simulink library "MultiModelToolbox"  (R2024b)
settings: Solver=VariableStepAuto  StartTime=0.0  StopTime=10.0  RelTol=1e-3
undefined symbols (not defined in the file): A, B, C, D, gravitationalAcceleration, MotorTorqueMax, roadB, roadC, roadD, roadE, roadSlope, stateSpace, Ts
libraries: $bdroot x5, autolibshared x1
settings Model: Creator=jdazo054  LastModifiedBy=jdazo054

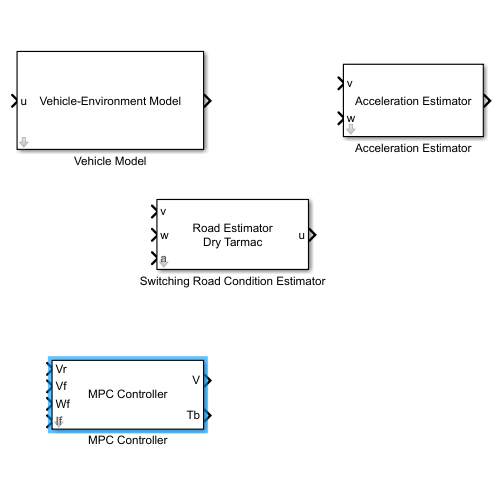
[thumbnail: Simulink's stored preview of the top-level diagram]
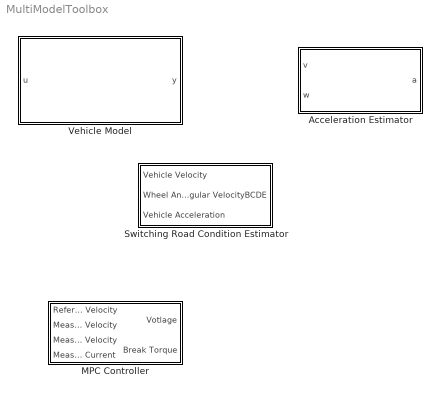
== system MultiModelToolbox ==
  Acceleration Estimator : Subsystem  mask{RoadCondition=Dry Tarmac, vehicleMass=1500, wheelInertia=0.8, wheelRadius=0.3, motorInertia=1, motorTorqueConstant=5, Clambda=0}
      mask prompts: RoadCondition "Road Condition"; vehicleMass "Vehicle Mass"; wheelInertia "Wheel Inertia"; wheelRadius "Wheel Radius"; motorInertia "Axle Inertia"; motorTorqueConstant "Torque Constant"
      mask TypeOptions RoadCondition: Dry Tarmac | Wet Tarmac | Snow | Ice
      mask DialogControl DescGroupVar Prompt: Acceleration Estimator
      mask DialogControl DescTextVar Prompt: This subsystem estimates vehicle acceleration using a linearized Pacejka tire model and Newton’s second law. Tire force is computed based on the selected road condition, which determines the Pacejka coefficients. The estimated force is divided by the user-defined vehicle mass to calculate acceleration. Road friction effects are implicitly modeled through the road type parameter.
      mask DialogControl RoadCondition Tooltip: Road surface type (affects traction and friction). Selects the corresponding coefficients (B, C, D, E) for the Pacejka Magic Formula used to compute linearized tire stiffness (Clambda). Options: Dry Tarmac, Wet Tarmac, Snow, Ice.
      mask DialogControl Container3 Prompt: Vehicle Parameters
      mask DialogControl vehicleMass Tooltip: Mass of the vehicle in kilograms (kg).
      mask DialogControl wheelInertia Tooltip: Moment of inertia of the wheel in kg·m².
      mask DialogControl wheelRadius Tooltip: Radius of the wheel in meters (m).
      mask DialogControl Container4 Prompt: Motor Parameters
      mask DialogControl motorInertia Tooltip: Moment of inertia of the motor rotor in kg·m².
      mask DialogControl motorTorqueConstant Tooltip: Motor torque constant in newton-meters per ampere (Nm/A).
      mask DialogControl Container5 Prompt: Invisible Parameters
      mask Display:
      | disp('Acceleration Estimator');
      | port_label('input', 1, 'v');
      | port_label('input', 2, 'w');
  MPC Controller : Subsystem  mask{Parameter1=0, stateSpace=stateSpace}
      mask prompts: Parameter1 "Prediction Horizon"
      mask DialogControl DescGroupVar Prompt: EV Model Predictive Controller
      mask DialogControl DescTextVar Prompt: This block implements a discrete-time linear Model Predictive Control (MPC) for set-point tracking of a 3-state, 1-input system.
      mask Display:
      | disp('MPC Controller');
      | port_label('input', 1, 'Vr');
      | port_label('input', 2, 'Vf');
      | port_label('input', 3, 'Wf');
      | port_label('input', 4, 'If');
      | port_label('output', 1, 'V');
      | port_label('output', 2, 'Tb');
  Switching Road Condition Estimator : Subsystem  mask{currentRoadIdx=1}
      mask Display:
      | % Display title
      | disp('Road Estimator\n');
      | 
      | currentRoadIdx = get_param(gcb, "currentRoadIdx");
      | 
      | % Display road label (use variable stored in mask or workspace)
      | switch currentRoadIdx
      |     case '1'
      |         disp('\nDry Tarmac');
      |     case '2'
      |         disp('\nWet Tarmac');
      |     case '3'
      |         disp('\nSnow');
      |     case '4'
      |         disp('\nIce');
      |     otherwise
      |         disp("\nUnknown");
      | end
      | port_label('input', 1, 'v');
      | port_label('input', 2, 'w');
      | port_label('input', 3, 'a');
      | port_label('output', 1, 'u');
  Vehicle Model : Subsystem  mask{RoadCondition=Dry Tarmac, vehicleMass=1500, wheelInertia=0.8, wheelRadius=0.3, motorInertia=1, motorResistance=0.1, motorTorqueConstant=5, motorInductance=0.005, motorBackEMFConstant=0.004, A_matrix=0, B_matrix=0, C_matrix=0, D_matrix=0}
      mask prompts: RoadCondition "Road Condition"; vehicleMass "Vehicle Mass"; wheelInertia "Wheel Inertia"; wheelRadius "Wheel Radius"; motorInertia "Axle Inertia"; motorResistance "Armature Resistance"; motorTorqueConstant "Torque Constant"; motorInductance "Armature Inductance"; motorBackEMFConstant "Armature EMF Constant"
      mask TypeOptions RoadCondition: Dry Tarmac | Wet Tarmac | Snow | Ice
      mask DialogControl DescGroupVar Prompt: Vehicle-Environment Model
      mask DialogControl DescTextVar Prompt: MATLAB/SIMULINK Model of a Vehicle. Designed for Longitudinal Road Friction Adaptive Control using Multi-Model Adaptive Estimators (MMAEs)
      mask DialogControl RoadCondition Tooltip: Road surface type (affects traction and friction). Selects the corresponding coefficients (B, C, D, E) for the Pacejka Magic Formula used to compute linearized tire stiffness (Clambda). Options: Dry Tarmac, Wet Tarmac, Snow, Ice.
      mask DialogControl Container3 Prompt: Vehicle Parameters
      mask DialogControl vehicleMass Tooltip: Mass of the vehicle in kilograms (kg).
      mask DialogControl wheelInertia Tooltip: Moment of inertia of the wheel in kg·m².
      mask DialogControl wheelRadius Tooltip: Radius of the wheel in meters (m).
      mask DialogControl Container4 Prompt: Motor Parameters
      mask DialogControl motorInertia Tooltip: Moment of inertia of the motor rotor in kg·m².
      mask DialogControl motorResistance Tooltip: Electrical resistance of the motor windings in ohms (Ω).
      mask DialogControl motorTorqueConstant Tooltip: Motor torque constant in newton-meters per ampere (Nm/A).
      mask DialogControl motorInductance Tooltip: Electrical inductance of the motor windings in henries (H).
      mask DialogControl motorBackEMFConstant Tooltip: Motor back EMF constant in volts per radian per second (V·s/rad).
      mask Display:
      | disp('Vehicle-Environment Model');
      | port_label('input', 1, 'u');

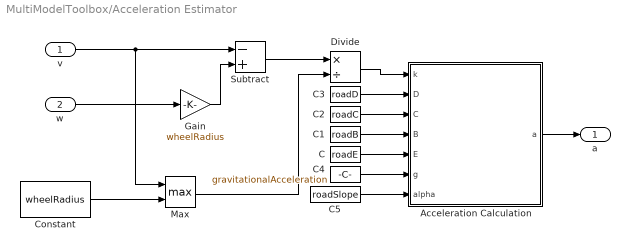
== system MultiModelToolbox/Acceleration Estimator ==
  v : Inport
  w : Inport  Port=2
  Acceleration Calculation : MATLAB Function  TreatAsAtomicUnit=on
  C : Constant  Value=roadE
  C1 : Constant  Value=roadB
  C2 : Constant  Value=roadC
  C3 : Constant  Value=roadD
  C4 : Constant  Value=gravitationalAcceleration
  C5 : Constant  Value=roadSlope
  Constant : Constant  Value=wheelRadius
  Divide : Product  Inputs=*/
  Gain : Gain  Gain=wheelRadius
  Max : MinMax  Function=max  Inputs=2
  Subtract : Sum  Inputs=-+
  a : Outport
  wires:
  Constant/1 -> Max/2
  v/1 -> Max/1, Subtract/1
  w/1 -> Gain/1
  Gain/1 -> Subtract/2
  Subtract/1 -> Divide/1
  Max/1 -> Divide/2
  Divide/1 -> Acceleration Calculation/1(k)
  C3/1 -> Acceleration Calculation/2(D)
  C2/1 -> Acceleration Calculation/3(C)
  C1/1 -> Acceleration Calculation/4(B)
  C/1 -> Acceleration Calculation/5(E)
  C4/1 -> Acceleration Calculation/6(g)
  C5/1 -> Acceleration Calculation/7(alpha)
  Acceleration Calculation/1(a) -> a/1

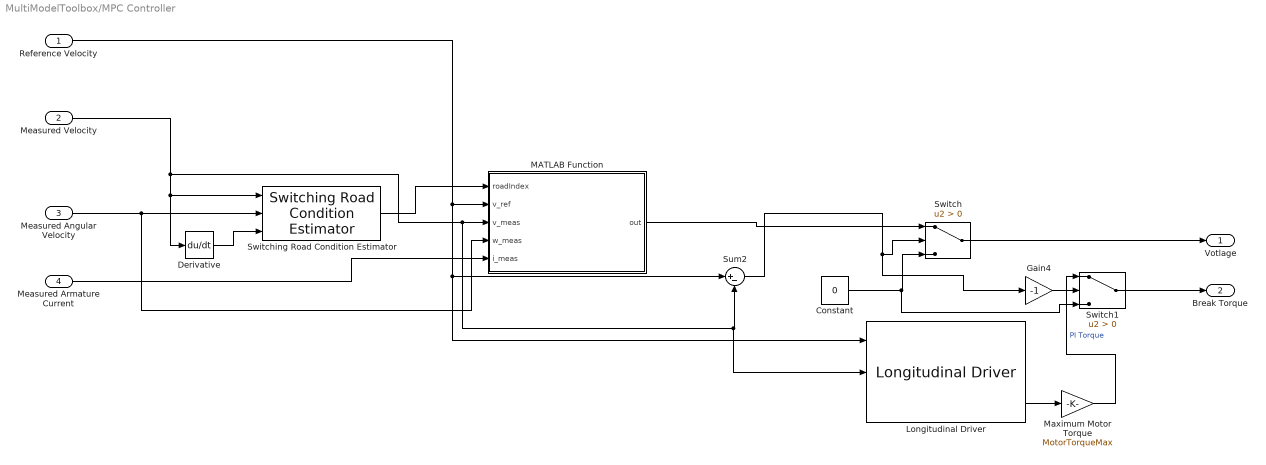
== system MultiModelToolbox/MPC Controller ==
  Reference Velocity : Inport
  Measured Velocity : Inport  Port=2
  Measured Angular Velocity : Inport  Port=3
  Measured Armature Current : Inport  Port=4
  Constant : Constant  Value=0
  Derivative : Derivative
  Gain4 : Gain  Gain=-1
  Longitudinal Driver : autolibshared/Longitudinal Driver  extAccelOvr=off  extDecelOvr=off  extAccelHld=off  extDecelHld=off  extAccelZero=off  extDecelZero=off  cntrlType=PI  shftType=None  velUnits=m/s  gearOut=off  Kp=8  Ki=2  Kff=.1  Kg=0  VehVelVec=[0 100]  KffVec=[.1 .1]  KpVec=[10 10]  KiVec=[5 5]  KgVec=[0 0]  m=1500  Kpt=3000  tau=.1  L=2  aR=200  bR=2.5  cR=.5  g=9.81  vnom=5  Kaw=1  tauerr=.01  tauPt=2  GearInit=0  tShift=.1  pdlVec=[0.1 0.4 0.5 0.9]  upShftTbl=[-1 12.9375 26.4375 39.9375 51.18749999999999 62.4375 72.84375 83.25;-1 16.3125 29.8125 43.3125 54.5624 65.8125 76.78125 87.75;-1 19.6875 33.1875 46.68749999999999 57.9375 69.1875 80.71875 92.25;-1 33 52.5 77.25 100.5 138.75 161.875 185]  dwnShftTbl=[1 9.5625 23.0625 36.5625 47.8125 59.0625 68.90625 78.75;1 12.9375 26.4375 39.9375 51.18749999999999 62.4375 72.84375 83.25;1 16.3125 29.8125 43.3125 54.562499 65.8125 76.78125 87.75;1 19.6875 33.1875 46.68749999999999 57.9375 69.1875 80.71875 92.25]  tClutch=.5  tRev=.5  tPark=120  aMode=2  UpGearVec="[0  1  2  3  4  5  6  7]"  DownGearVec="[1  2  3  4  5  6  7  8]"
      settings: LibrarySourceBlock=vehdynlibdriver/Longitudinal Driver
  MATLAB Function : MATLAB Function  TreatAsAtomicUnit=on  SystemSampleTime=Ts
  Maximum Motor Torque : Gain  Gain=MotorTorqueMax
  Sum2 : Sum  Inputs=|+-
  Switch : Switch  Criteria=u2 > Threshold  SaturateOnIntegerOverflow=off  InputSameDT=off
  Switch1 : Switch  Criteria=u2 > Threshold  SaturateOnIntegerOverflow=off  InputSameDT=off
  Switching Road Condition Estimator : $bdroot/Switching Road Condition Estimator  currentRoadIdx=1
  Votlage : Outport
  Break Torque : Outport  Port=2
  wires:
  Reference Velocity/1 -> Longitudinal Driver/1, Sum2/1, MATLAB Function/2(v_ref)
  Measured Angular Velocity/1 -> MATLAB Function/4(w_meas), Switching Road Condition Estimator/2
  Measured Velocity/1 -> Longitudinal Driver/2, Sum2/2, MATLAB Function/3(v_meas), Derivative/1, Switching Road Condition Estimator/1
  Switching Road Condition Estimator/1 -> MATLAB Function/1(roadIndex)
  Derivative/1 -> Switching Road Condition Estimator/3
  MATLAB Function/1(out) -> Switch/1
  Measured Armature Current/1 -> MATLAB Function/5(i_meas)
  Switch/1 -> Votlage/1
  Longitudinal Driver/3 -> Maximum Motor Torque/1
  Constant/1 -> Switch1/3, Switch/3
  Maximum Motor Torque/1 -> Switch1/1  "PI Torque"
  Sum2/1 -> Gain4/1, Switch/2
  Gain4/1 -> Switch1/2
  Switch1/1 -> Break Torque/1

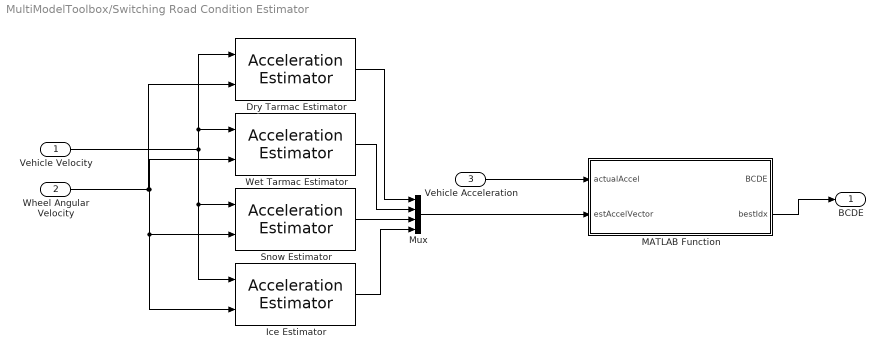
== system MultiModelToolbox/Switching Road Condition Estimator ==
  Vehicle Velocity : Inport
  Wheel Angular Velocity : Inport  Port=2
  Vehicle Acceleration : Inport  Port=3
  Dry Tarmac Estimator : $bdroot/Acceleration Estimator  RoadCondition=Dry Tarmac  vehicleMass=1500  wheelInertia=0.8  wheelRadius=0.3  motorInertia=1  motorTorqueConstant=5  Clambda=0
      link override Acceleration Calculation: SystemSampleTime=-1
  Ice Estimator : $bdroot/Acceleration Estimator  RoadCondition=Ice  vehicleMass=1500  wheelInertia=0.8  wheelRadius=0.3  motorInertia=1  motorTorqueConstant=5  Clambda=0
  MATLAB Function : MATLAB Function  TreatAsAtomicUnit=on
  Mux : Mux
  Snow Estimator : $bdroot/Acceleration Estimator  RoadCondition=Snow  vehicleMass=1500  wheelInertia=0.8  wheelRadius=0.3  motorInertia=1  motorTorqueConstant=5  Clambda=0
  Wet Tarmac Estimator : $bdroot/Acceleration Estimator  RoadCondition=Wet Tarmac  vehicleMass=1500  wheelInertia=0.8  wheelRadius=0.3  motorInertia=1  motorTorqueConstant=5  Clambda=0
  BCDE : Outport
  wires:
  Vehicle Velocity/1 -> Ice Estimator/1, Snow Estimator/1, Dry Tarmac Estimator/1, Wet Tarmac Estimator/1
  Wheel Angular Velocity/1 -> Ice Estimator/2, Snow Estimator/2, Wet Tarmac Estimator/2, Dry Tarmac Estimator/2
  Dry Tarmac Estimator/1 -> Mux/1
  Wet Tarmac Estimator/1 -> Mux/2
  Snow Estimator/1 -> Mux/3
  Ice Estimator/1 -> Mux/4
  Mux/1 -> MATLAB Function/2(estAccelVector)
  Vehicle Acceleration/1 -> MATLAB Function/1(actualAccel)
  MATLAB Function/2(bestIdx) -> BCDE/1

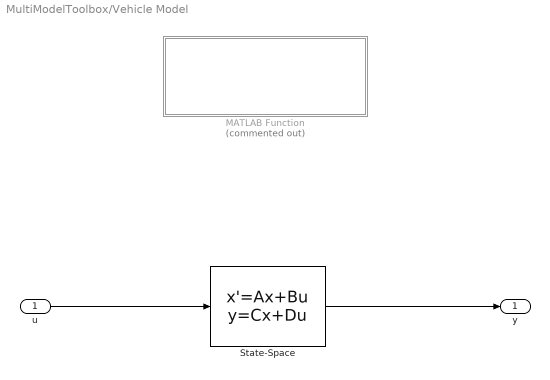
== system MultiModelToolbox/Vehicle Model ==
  u : Inport
  MATLAB Function : MATLAB Function  Commented=on  TreatAsAtomicUnit=on
  State-Space : StateSpace  A=A_matrix  B=B_matrix  C=C_matrix  D=D_matrix  InitialCondition=0
  y : Outport
  wires:
  u/1 -> State-Space/1
  State-Space/1 -> y/1

== matlab function MultiModelToolbox/Acceleration Estimator/Acceleration Calculation ==
  data: k input; a output; D input; C input; B input; E input; g input; alpha input
function a = PacejkaFormula(k, D, C, B, E, g, alpha)
    
    % Compute acceleration
    num_wheels = 2;
    ux = D * sin(C * atan(B * k - E * (B * k - atan(B * k))));
    a = num_wheels * 1 * cos(alpha) * ux;

== matlab function MultiModelToolbox/Vehicle Model/MATLAB Function ==
  data: B parameter; C parameter; D parameter; A parameter
function GenerateStateSpaceMatrices(B, C, D, A)
%#codegen

% Get parameters from the block mask
roadCondition        = get_param(gcb, 'RoadCondition'); % e.g. 'Dry Tarmac'
vehicleMass          = str2double(get_param(gcb, 'vehicleMass'));         
wheelInertia         = str2double(get_param(gcb, 'wheelInertia'));        
wheelRadius          = str2double(get_param(gcb, 'wheelRadius'));         
motorInertia         = str2double(get_param(gcb, 'motorInertia'));        
motorResistance      = str2double(get_param(gcb, 'motorResistance'));     
motorInductance      = str2double(get_param(gcb, 'motorInductance'));     
motorTorqueConstant  = str2double(get_param(gcb, 'motorTorqueConstant')); 
motorBackEMFConstant = str2double(get_param(gcb, 'motorBackEMFConstant'));

% Gravity constant
g = 9.81;

% Set Magic Formula Coefficients based on Road Condition    
switch roadCondition
    case 'Dry Tarmac'
        roadB = 10; roadC = 1.9; roadD = 1; roadE = 0.97;
    case 'Wet Tarmac'
        roadB = 12; roadC = 2.3; roadD = 0.82; roadE = 1;
    case 'Snow'
        roadB = 5;  roadC = 2;   roadD = 0.3;  roadE = 1;
    case 'Ice'
        roadB = 4;  roadC = 2;   roadD = 0.1;  roadE = 1;
    otherwise
        roadB = 10; roadC = 1.9; roadD = 1; roadE = 0.97;
end

% Compute linearized slip stiffness based of the derivative
Clambda = roadB*roadC*roadD

A = [
    (- 4* Clambda * gravitationalAcceleration * cos(roadSlope)) / wheelRadius - C1 / vehicleMass, 4*Clambda * gravitationalAcceleration * cos(roadSlope), 0;
    (4*Clambda * gravitationalAcceleration * cos(roadSlope)) / (motorInertia + wheelInertia), - (4*Clambda * wheelRadius * vehicleMass * gravitationalAcceleration * cos(roadSlope)) / (motorInertia + wheelInertia), motorTorqueConstant / (motorInertia + wheelInertia);
    0, -motorBackEMFConstant / motorInductance, -motorResistance / motorInductance
];

% Define B matrix with input voltage (Vin)
B = [
    0;
    0;
    1 / motorInductance
];

% Output matrix (only velocity is measured)
C = [1 0 0]; 
D = 0;

== matlab function MultiModelToolbox/Switching Road Condition Estimator/MATLAB Function ==
  settings: updateMethod=DISCRETE
  data: actualAccel input; BCDE output; estAccelVector input; bestIdx output
function [BCDE, bestIdx] = fcn(actualAccel, estAccelVector)
% Inputs:
%   actualAccel     - scalar (latest measured acceleration)
%   estAccelVector  - 4×1 vector (latest estimated acceleration for each road condition)
% Outputs:
%   BCDE            - 1×4 vector: [B C D E] for best-fit road
%   bestIdx         - integer: index of best-fit road condition

    % --- Parameters ---
    windowSize = 1000;  % Moving average window size (adjustable)

    % Define road surface Pacejka parameters: [B C D E]
    params = [
        10, 1.9, 1.00, 0.97;  % Dry
        12, 2.3, 0.82, 1.00;  % Wet
        5,  2.0, 0.30, 1.00;  % Snow
        4,  2.0, 0.10, 1.00   % Ice
    ];

    numConditions = size(params, 1);

    % --- Persistent Error History Buffer ---
    persistent errHist
    if isempty(errHist)
        errHist = zeros(numConditions, windowSize);
    end

    % --- Update Buffer with New Squared Errors ---
    for i = 1:numConditions
        %fprintf("Road Condition: %d", i);
        err = actualAccel - estAccelVector(i);
        %fprintf("Error: %d", err);
        errHist(i, :) = [errHist(i, 2:end), err^2];  % Shift left, append new
    end

    % --- Compute Smoothed Error (Moving Average) ---
    avgError = mean(errHist, 2);  % 4×1 vector

    % --- Find Best Matching Road Condition ---
    [~, bestIdx] = min(avgError);
    BCDE = params(bestIdx, :);
end

== matlab function MultiModelToolbox/MPC Controller/MATLAB Function ==
  data: roadIndex input; out output; v_ref input; v_meas input; w_meas input; i_meas input; stateSpace parameter
function out = lmpc_step(roadIndex, v_ref, v_meas, w_meas, i_meas, stateSpace)
% LMPC_STEP  One-step linear MPC with condensed QP formulation.
% Inputs:
%   roadIndex : integer in {1=dry, 2=wet, 3=snow, 4=ice}
%   v_ref     : current reference velocity [m/s] (assumed constant over horizon)
%   v_meas    : measured vehicle velocity [m/s]
%

    %===========================================================
    % 0) MPC Controller Parameter Definition
    %===========================================================

    switch roadIndex
        case 1
            A_matrix = stateSpace.dry_tarmac.A;
            B_matrix = stateSpace.dry_tarmac.B;
        case 2
            A_matrix = stateSpace.wet_tarmac.A;
            B_matrix = stateSpace.wet_tarmac.B;
        case 3
            A_matrix = stateSpace.snow.A;
            B_matrix = stateSpace.snow.B;
        case 4
            A_matrix = stateSpace.ice.A;
            B_matrix = stateSpace.ice.B;
        otherwise
            A_matrix = stateSpace.dry_tarmac.A;
            B_matrix = stateSpace.dry_tarmac.B;
    end

    % Simulation parameters
    prediction_horizon = 5;          % MPC prediction horizon (N)
    state_dimension = 3;             % Number of system states (n)
    input_dimension = 1;             % Number of system inputs (m)

    % Cost function weighting matrices
    Q_state_weight = diag([50, 1e-12, 1e-12]);      % State penalty matrix (Q)
    Q_terminal_weight = Q_state_weight;        % Terminal state penalty (QN)
    R_input_weight = 1e-6;     % Input penalty matrix (R)

    % Reference signal computation (set point)
    x_reference = [v_ref; 0; 0]; % Desired state
    u_reference = pinv(B_matrix) * (eye(state_dimension)-A_matrix) * x_reference;

    % State constraints (Fx * x <= gx)
    Fx = [1 0 0; -1 0 0; 0 1 0; 0 -1 0; 0 0 1; 0 0 -1];                 % State constraint matrix
    gx = [10; 10; 10; 10; 10 ; 10] - Fx * x_reference;    % State constraint bounds (shifted by reference)

    % Input constraints (Fu * u <= gu)
    Fu = [1; -1];                                % Input constraint matrix
    gu = [10; 10] - Fu * u_reference;              % Input constraint bounds (shifted by reference)
    

    %===========================================================
    % 1) Lifted prediction matrices AX, BU (for states) and Oy
    %===========================================================

    % Lifted state/input matrices
    x_initial = [v_meas; w_meas; i_meas];

    X_prediction = zeros(state_dimension*(prediction_horizon+1),1); 
    X_prediction(1:state_dimension,1) = x_initial - x_reference;  % Predicted state trajectory

    U_prediction = zeros(input_dimension*prediction_horizon,1); % Predicted inputs


    % Decision vector for optimizer (contains states & inputs)
    z_decision = [X_prediction; U_prediction];


    % Build AX (state evolution) and BU (control influence)

    AX = zeros(state_dimension*(prediction_horizon+1), state_dimension);
    BU = zeros(state_dimension*(prediction_horizon+1), input_dimension*prediction_horizon);
    for i = 1:prediction_horizon+1
        AX((i-1)*state_dimension+1:i*state_dimension,:) = A_matrix^(i-1);
    end
    
    for i = 1:prediction_horizon+1
        for j = 1:prediction_horizon
            if i > j
                BU((i-1)*state_dimension+1:i*state_dimension, ...
                   (j-1)*input_dimension+1:j*input_dimension) = ...
                   A_matrix^(i-j-1)*B_matrix;
            else
                BU((i-1)*state_dimension+1:i*state_dimension, ...
                   (j-1)*input_dimension+1:j*input_dimension) = zeros(state_dimension,input_dimension);
            end    
        end
    end


    % Extended weighting matrices for optimization


    QX = []; 
    RU = [];
    FX = []; gX = []; 
    FU = []; gU = [];
    
    % Preallocate with fixed sizes
    QX = zeros(state_dimension*(prediction_horizon+1), state_dimension*(prediction_horizon+1));
    RU = zeros(input_dimension*(prediction_horizon), input_dimension*(prediction_horizon));
    FX = zeros(size(Fx,1)*(prediction_horizon+1), size(Fx,2)*(prediction_horizon+1));
    gX = zeros(size(gx,1)*(prediction_horizon+1), 1);
    FU = zeros(size(Fu,1)*(prediction_horizon), size(Fu,2)*(prediction_horizon));
    gU = zeros(size(gu,1)*(prediction_horizon), 1);
    
    % Fill block diagonals for stage cost
    for i = 1:prediction_horizon-1
        % Q blocks
        idx = (i-1)*state_dimension+1 : i*state_dimension;
        QX(idx,idx) = Q_state_weight;
    
        % R blocks
        idxu = (i-1)*input_dimension+1 : i*input_dimension;
        RU(idxu,idxu) = R_input_weight;
    
        % Fx and gx
        idfx = (i-1)*size(Fx,1)+1 : i*size(Fx,1);
        idxx = (i-1)*size(Fx,2)+1 : i*size(Fx,2);
        FX(idfx, idxx) = Fx;
        gX(idfx) = gx;
    
        % Fu and gu
        idfu = (i-1)*size(Fu,1)+1 : i*size(Fu,1);
        iduu = (i-1)*size(Fu,2)+1 : i*size(Fu,2);
        FU(idfu, iduu) = Fu;
        gU(idfu) = gu;
    end
    
    % Final QN block
    idx = (prediction_horizon-1)*state_dimension+1 : prediction_horizon*state_dimension;
    QX(idx,idx) = Q_terminal_weight;
    
    % Final Fx and gx
    idfx = (prediction_horizon-1)*size(Fx,1)+1 : prediction_horizon*size(Fx,1);
    idxx = (prediction_horizon-1)*size(Fx,2)+1 : prediction_horizon*size(Fx,2);
    FX(idfx, idxx) = Fx;
    gX(idfx) = gx;
    
    % Build H
    Hessian = blkdiag(QX, RU);

    %===========================================================
    % 2) Cost: J = (Y - r)'Qy_blk(Y - r) + U'RU
    %===========================================================

   current_state = x_initial - x_reference;  

   % Constraints
   inequality_matrix = blkdiag(FX, FU); 
   inequality_vector = [gX; gU];
   equality_matrix = [eye((prediction_horizon+1)*state_dimension), -BU];
   equality_vector = AX * current_state;

   % Solve QP (fmincon used here)

   f = zeros(size(Hessian,1),1);
    
   options = optimoptions('quadprog', 'Algorithm', 'active-set', 'Display', 'off');

   z_solution = quadprog(Hessian, f, inequality_matrix, inequality_vector, equality_matrix, equality_vector, [], [], z_decision, options);


   % Warm start: use last solution as initial guess
   z_decision = z_solution;

   out = z_solution((prediction_horizon+1)*state_dimension+1 : ...
                       (prediction_horizon+1)*state_dimension+input_dimension, 1);
